simulink model "simulink_model"  (R2023b)
settings: Solver=VariableStepAuto  StartTime=0.0  StopTime=100  RelTol=1e-3
undefined symbols (not defined in the file): sys_mimo
settings Model: Creator=kaleb  LastModifiedBy=kaleb

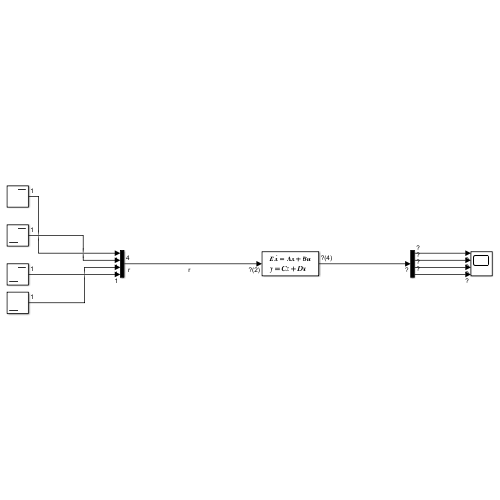
[thumbnail: Simulink's stored preview of the top-level diagram]
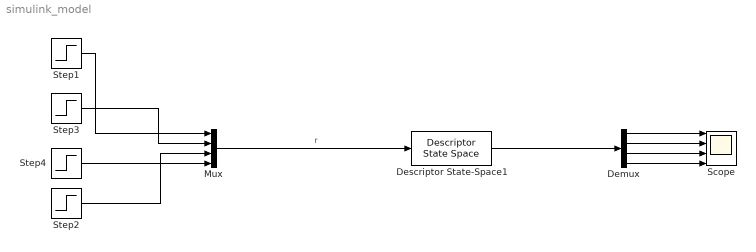
== system simulink_model ==
  Demux : Demux
  Descriptor State-Space1 : DescriptorStateSpace  E=eye(4)  A=sys_mimo.A  B=sys_mimo.B  C=sys_mimo.C  D=sys_mimo.D  DirectFeedthrough=False
  Mux : Mux
  Scope : Scope  NumInputPorts=4
  Step1 : Step  After=1*pi/180  SampleTime=0
  Step2 : Step  After=0.1  SampleTime=0
  Step3 : Step  After=1*pi/180  SampleTime=0
  Step4 : Step  After=1*pi/180  SampleTime=0
  wires:
  Step2/1 -> Mux/3
  Step1/1 -> Mux/1
  Descriptor State-Space1/1 -> Demux/1
  Demux/1 -> Scope/1
  Demux/2 -> Scope/2
  Demux/3 -> Scope/3
  Demux/4 -> Scope/4
  Mux/1 -> Descriptor State-Space1/1  "r"
  Step3/1 -> Mux/2
  Step4/1 -> Mux/4
